simulink model "nonliner_saturation"  (R2019a)
settings: Solver=VariableStepAuto  StartTime=0.0  StopTime=40  RelTol=1e-3
libraries: simulink x3
settings Model: Creator=Mohamed Nofal  LastModifiedBy=Mohamed Nofal

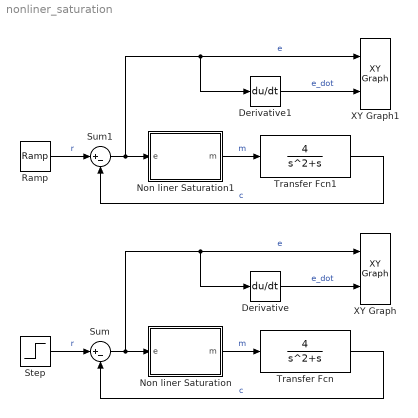
== system nonliner_saturation ==
  Derivative : Derivative
  Derivative1 : Derivative
  Non liner Saturation : MATLAB Function  TreatAsAtomicUnit=on
  Non liner Saturation1 : MATLAB Function  TreatAsAtomicUnit=on
  Ramp : simulink/Sources/Ramp  slope=0.7  start=0  InitialOutput=0
  Step : Step
  Sum : Sum  Inputs=|+-
  Sum1 : Sum  Inputs=|+-
  Transfer Fcn : TransferFcn  Numerator=[4]  Denominator=[1,1,0]
  Transfer Fcn1 : TransferFcn  Numerator=[4]  Denominator=[1,1,0]
  XY Graph : simulink/Sinks/XY Graph  xmin=-1  xmax=1  ymin=-1  ymax=1  st=.1
  XY Graph1 : simulink/Sinks/XY Graph  xmin=-1  xmax=1  ymin=-1  ymax=1  st=.1
  wires:
  Non liner Saturation/1(m) -> Transfer Fcn/1  "m"
  Sum/1 -> Non liner Saturation/1(e), Derivative/1, XY Graph/1  "e"
  Transfer Fcn/1 -> Sum/2  "c"
  Step/1 -> Sum/1  "r"
  Derivative/1 -> XY Graph/2  "e_dot"
  Derivative1/1 -> XY Graph1/2  "e_dot"
  Ramp/1 -> Sum1/1  "r"
  Transfer Fcn1/1 -> Sum1/2  "c"
  Sum1/1 -> XY Graph1/1, Derivative1/1, Non liner Saturation1/1(e)  "e"
  Non liner Saturation1/1(m) -> Transfer Fcn1/1  "m"

== matlab function nonliner_saturation/Non liner Saturation1 ==
  data: e input; m output
function m = fcn(e)
if e<-0.2
    m=-0.2;
elseif e>0.2
    m=0.2;
else 
    m=e;
end
m=m ;

== matlab function nonliner_saturation/Non liner Saturation ==
  data: e input; m output
function m = fcn(e)
if e<-0.2
    m=-0.2;
elseif e>0.2
    m=0.2;
else 
    m=e;
end
m=m ;
